simulink model "washout"  (R2018b)
settings: Solver=VariableStepAuto  StartTime=0.0  StopTime=Time(end)  RelTol=1e-3
values from neighbouring files (symbols this model uses):
  Cf = 80000    [init.m]
  Cr = 90000    [init.m]
  dG = 0.05    [init.m]
  g = 9.81    [init.m]
  lf = cog_x*L    (= 0.70125)    [init.m]
  lr = (1-cog_x)*L    (= 2.10375)    [init.m]
  mass = 1905    [init.m]
  Ratio = 10    [init.m]
  rx = 30e-2    (= 0.3)    [init.m]
  swaThreshold = 5    [init.m]
  T0 = 0.3    [init.m]
  TH = 0.1    [init.m]
  TTh = 0.1    [init.m]
  vxThreshold = 0.5    [init.m]
  xC = 0    [init.m]
  xG = 0.01    [init.m]
  yawThreshold = 0.1    [init.m]
undefined symbols (not defined in the file or in its folder): T
libraries: simulink_extras x3, dsparch4 x1
settings Model: Creator=carl  LastModifiedBy=carl

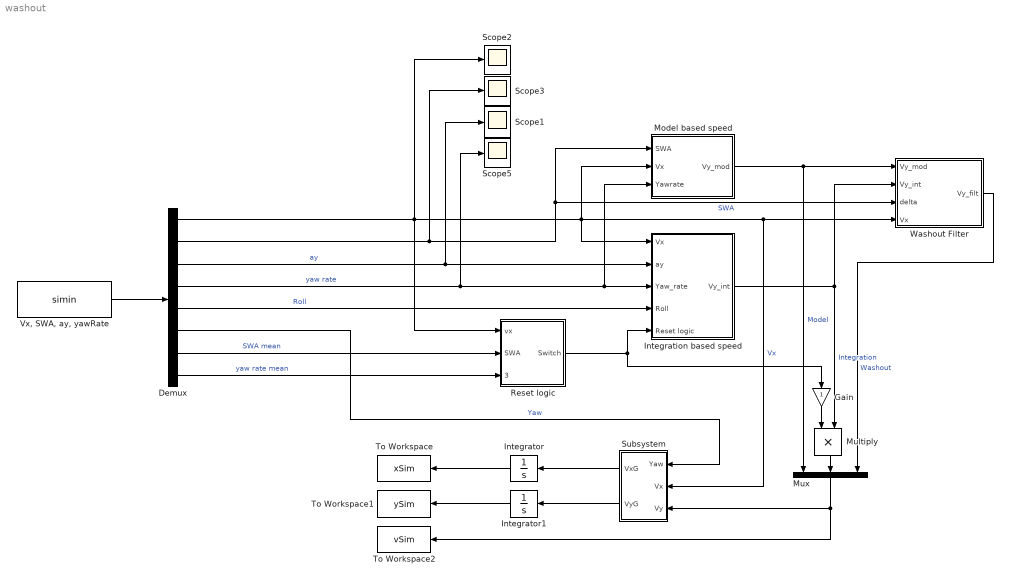
== system washout ==
  Demux : Demux  Outputs=8
  Gain : Gain
  Integration based speed : Subsystem
  Integrator : Integrator
  Integrator1 : Integrator
  Model based speed : Subsystem
  Multiply : Product
  Mux : Mux  Inputs=3
  Reset logic : Subsystem
  Scope{1..3,5} (4 alike) : Scope
  Subsystem : Subsystem
  To Workspace : ToWorkspace  VariableName=xSim  SaveFormat=Timeseries  SampleTime=-1
  To Workspace1 : ToWorkspace  VariableName=ySim  SaveFormat=Timeseries  SampleTime=-1
  To Workspace2 : ToWorkspace  VariableName=vSim  SaveFormat=Timeseries  SampleTime=-1
  "Vx, SWA, ay, yawRate" : FromWorkspace  VariableName=simin  SampleTime=0
  Washout Filter : Subsystem
  wires:
  Demux/3 -> Scope1/1, Integration based speed/2(ay)  "ay"
  Model based speed/1(Vy_mod) -> Mux/1, Washout Filter/1(Vy_mod)  "Model"
  Demux/2 -> Scope3/1, Washout Filter/3(delta), Model based speed/1(SWA)  "SWA"
  Demux/1 -> Reset logic/1(vx), Integration based speed/1(Vx), Washout Filter/4(Vx), Subsystem/2(Vx), Model based speed/2(Vx), Scope2/1  "Vx"
  Integration based speed/1(Vy_int) -> Multiply/2, Washout Filter/2(Vy_int)  "Integration"
  Demux/4 -> Model based speed/3(Yawrate), Integration based speed/3(Yaw_rate), Scope5/1  "yaw rate"
  Washout Filter/1(Vy_filt) -> Mux/3  "Washout"
  Integrator/1 -> To Workspace/1
  "Vx, SWA, ay, yawRate"/1 -> Demux/1
  Integrator1/1 -> To Workspace1/1
  Subsystem/2(VyG) -> Integrator1/1
  Subsystem/1(VxG) -> Integrator/1
  Demux/5 -> Integration based speed/4(Roll)  "Roll"
  Demux/6 -> Subsystem/1(Yaw)  "Yaw"
  Mux/1 -> To Workspace2/1, Subsystem/3(Vy)
  Reset logic/1(Switch) -> Gain/1, Integration based speed/5(Reset logic)
  Multiply/1 -> Mux/2
  Gain/1 -> Multiply/1
  Demux/7 -> Reset logic/2(SWA)  "SWA mean"
  Demux/8 -> Reset logic/3(yawrate)  "yaw rate mean"

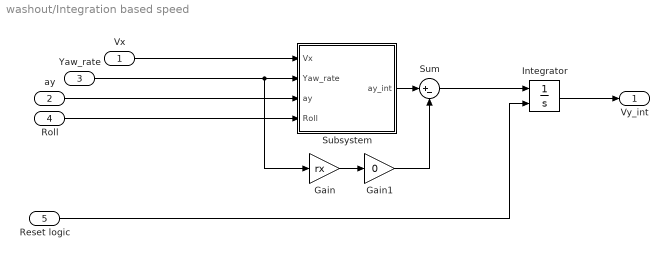
== system washout/Integration based speed ==
  Vx : Inport
  ay : Inport  Port=2
  Yaw_rate : Inport  Port=3
  Roll : Inport  Port=4
  Reset logic : Inport  Port=5
  Gain : Gain  Gain=rx
  Gain1 : Gain  Gain=0
  Integrator : Integrator  ExternalReset=rising
  Subsystem : Subsystem
  Sum : Sum  Inputs=|+-
  Vy_int : Outport
  wires:
  Vx/1 -> Subsystem/1(Vx)
  Yaw_rate/1 -> Gain/1, Subsystem/2(Yaw_rate)
  ay/1 -> Subsystem/3(ay)
  Subsystem/1(ay_int) -> Sum/1
  Roll/1 -> Subsystem/4(Roll)
  Gain/1 -> Gain1/1
  Gain1/1 -> Sum/2
  Sum/1 -> Integrator/1
  Integrator/1 -> Vy_int/1
  Reset logic/1 -> Integrator/2

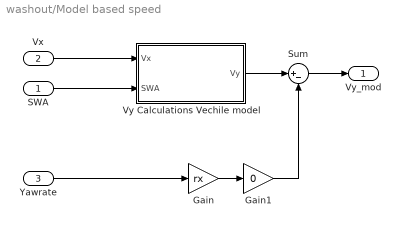
== system washout/Model based speed ==
  SWA : Inport
  Vx : Inport  Port=2
  Yawrate : Inport  Port=3
  Gain : Gain  Gain=rx
  Gain1 : Gain  Gain=0
  Sum : Sum  Inputs=|+-
  Vy Calculations Vechile model : Subsystem
  Vy_mod : Outport
  wires:
  Vx/1 -> Vy Calculations Vechile model/1(Vx)
  Vy Calculations Vechile model/1(Vy) -> Sum/1
  SWA/1 -> Vy Calculations Vechile model/2(SWA)
  Sum/1 -> Vy_mod/1
  Yawrate/1 -> Gain/1
  Gain/1 -> Gain1/1
  Gain1/1 -> Sum/2

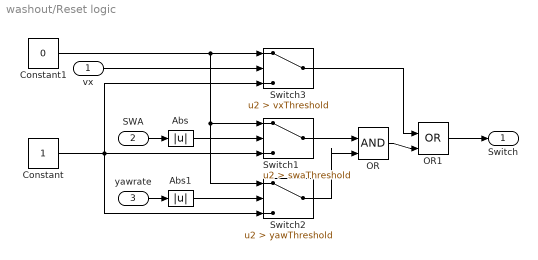
== system washout/Reset logic ==
  vx : Inport
  SWA : Inport  Port=2
  yawrate : Inport  Port=3
  Abs : Abs
  Abs1 : Abs
  Constant : Constant
  Constant1 : Constant  Value=0
  OR : Logic  IconShape=distinctive  AllPortsSameDT=off  OutDataTypeStr=boolean
  OR1 : Logic  Operator=OR  IconShape=distinctive  AllPortsSameDT=off  OutDataTypeStr=boolean
  Switch1 : Switch  Criteria=u2 > Threshold  Threshold=swaThreshold
  Switch2 : Switch  Criteria=u2 > Threshold  Threshold=yawThreshold
  Switch3 : Switch  Criteria=u2 > Threshold  Threshold=vxThreshold
  Switch : Outport
  wires:
  OR1/1 -> Switch/1
  Switch2/1 -> OR/2
  Constant/1 -> Switch1/3, Switch3/3, Switch2/3
  Abs/1 -> Switch1/2
  SWA/1 -> Abs/1
  yawrate/1 -> Abs1/1
  OR/1 -> OR1/2
  Switch1/1 -> OR/1
  Switch3/1 -> OR1/1
  Constant1/1 -> Switch1/1, Switch2/1, Switch3/1
  Abs1/1 -> Switch2/2
  vx/1 -> Switch3/2

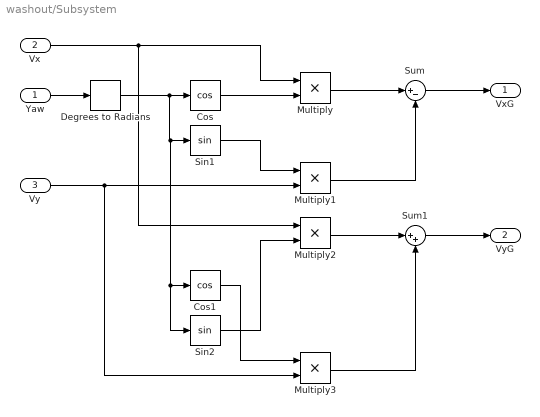
== system washout/Subsystem ==
  Yaw : Inport
  Vx : Inport  Port=2
  Vy : Inport  Port=3
  Cos : Trigonometry  Operator=cos
  Cos1 : Trigonometry  Operator=cos
  Degrees to Radians : simulink_extras/Transformations/Degrees to Radians
  Multiply{,1..3} (4 alike) : Product
  Sin1 : Trigonometry
  Sin2 : Trigonometry
  Sum : Sum  Inputs=|+-
  Sum1 : Sum  Inputs=|++
  VxG : Outport
  VyG : Outport  Port=2
  wires:
  Multiply/1 -> Sum/1
  Cos/1 -> Multiply/2
  Sin1/1 -> Multiply1/1
  Multiply1/1 -> Sum/2
  Sum/1 -> VxG/1
  Multiply2/1 -> Sum1/1
  Vx/1 -> Multiply2/1, Multiply/1
  Multiply3/1 -> Sum1/2
  Vy/1 -> Multiply1/2, Multiply3/2
  Sum1/1 -> VyG/1
  Sin2/1 -> Multiply2/2
  Cos1/1 -> Multiply3/1
  Yaw/1 -> Degrees to Radians/1
  Degrees to Radians/1 -> Sin2/1, Cos1/1, Sin1/1, Cos/1

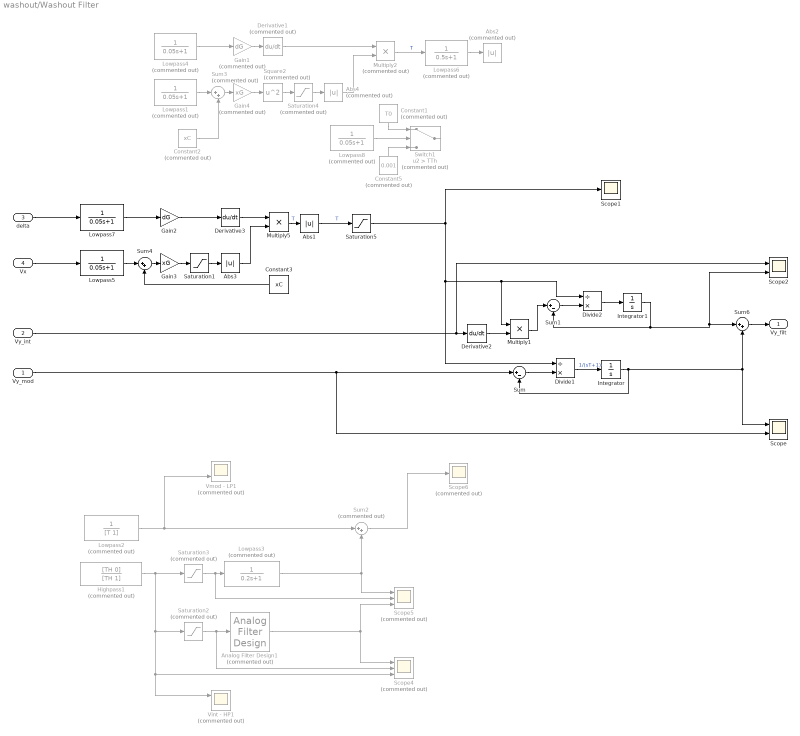
== system washout/Washout Filter ==
  Vy_mod : Inport
  Vy_int : Inport  Port=2
  delta : Inport  Port=3
  Vx : Inport  Port=4
  Abs1 : Abs
  Abs2 : Abs  Commented=on
  Abs3 : Abs
  Abs4 : Abs  Commented=on
  Analog Filter Design1 : dsparch4/Analog Filter Design  Commented=on  method=Butterworth  filttype=Lowpass  N=7  Wlo=8  Whi=80  Rp=2  Rs=40
  Constant1 : Constant  Commented=on  Value=T0
  Constant2 : Constant  Commented=on  Value=xC
  Constant3 : Constant  Value=xC
  Constant5 : Constant  Commented=on  Value=0.001
  Derivative1 : Derivative  Commented=on
  Derivative2 : Derivative
  Derivative3 : Derivative
  Divide1 : Product  Inputs=/*
  Divide2 : Product  Inputs=/*
  Gain1 : Gain  Commented=on  Gain=dG
  Gain2 : Gain  Gain=dG
  Gain3 : Gain  Gain=xG
  Gain4 : Gain  Commented=on  Gain=xG
  Highpass1 : TransferFcn  Commented=on  Numerator=[TH 0]  Denominator=[TH 1]
  Integrator : Integrator
  Integrator1 : Integrator
  Lowpass1 : TransferFcn  Commented=on  Denominator=[0.05 1]
  Lowpass2 : TransferFcn  Commented=on  Denominator=[T 1]
  Lowpass3 : TransferFcn  Commented=on  Denominator=[0.2 1]
  Lowpass4 : TransferFcn  Commented=on  Denominator=[0.05 1]
  Lowpass5 : TransferFcn  Denominator=[0.05 1]
  Lowpass6 : TransferFcn  Commented=on  Denominator=[0.5 1]
  Lowpass7 : TransferFcn  Denominator=[0.05 1]
  Lowpass8 : TransferFcn  Commented=on  Denominator=[0.05 1]
  Multiply1 : Product
  Multiply2 : Product  Commented=on
  Multiply5 : Product
  Saturation1 : Saturate  UpperLimit=2  LowerLimit=0
  Saturation2 : Saturate  Commented=on  UpperLimit=1  LowerLimit=-1
  Saturation3 : Saturate  Commented=on  UpperLimit=1  LowerLimit=-1
  Saturation4 : Saturate  Commented=on  UpperLimit=2  LowerLimit=0
  Saturation5 : Saturate  UpperLimit=T0  LowerLimit=0.01
  Scope : Scope  NumInputPorts=2
  Scope1 : Scope
  Scope2 : Scope  NumInputPorts=2
  Scope4 : Scope  Commented=on  NumInputPorts=3
  Scope5 : Scope  Commented=on  NumInputPorts=3
  Scope6 : Scope  Commented=on
  Square2 : Math  Commented=on  Operator=square  SaturateOnIntegerOverflow=on
  Sum : Sum  Inputs=|+-
  Sum1 : Sum  Inputs=|+-
  Sum2 : Sum  Commented=on  Inputs=|++
  Sum3 : Sum  Commented=on  Inputs=|++
  Sum4 : Sum  Inputs=|++
  Sum6 : Sum  Inputs=|++
  Switch1 : Switch  Commented=on  Criteria=u2 > Threshold  Threshold=TTh
  Vint - HP1 : Scope  Commented=on  NumInputPorts=2
  Vmod - LP1 : Scope  Commented=on  NumInputPorts=2
  Vy_filt : Outport
  wires:
  Saturation3/1 -> Lowpass3/1, Scope5/2
  Saturation2/1 -> Analog Filter Design1/1, Scope4/2
  Analog Filter Design1/1 -> Scope5/3, Scope4/1
  Lowpass3/1 -> Sum2/2, Scope5/1
  Lowpass2/1 -> Sum2/1, Vmod - LP1/2
  Sum2/1 -> Scope6/1
  Highpass1/1 -> Vint - HP1/1, Scope4/3, Saturation2/1, Saturation3/1
  Constant3/1 -> Sum4/2
  Sum4/1 -> Gain3/1
  Saturation1/1 -> Abs3/1
  Gain3/1 -> Saturation1/1
  Multiply5/1 -> Abs1/1  "T"
  Abs3/1 -> Multiply5/2
  Lowpass5/1 -> Sum4/1
  Derivative3/1 -> Multiply5/1
  Lowpass7/1 -> Gain2/1
  Gain2/1 -> Derivative3/1
  Gain1/1 -> Derivative1/1
  Lowpass4/1 -> Gain1/1
  Derivative1/1 -> Multiply2/1
  Lowpass6/1 -> Abs2/1
  Lowpass1/1 -> Sum3/1
  Abs4/1 -> Multiply2/2
  Multiply2/1 -> Lowpass6/1  "T"
  Gain4/1 -> Square2/1
  Square2/1 -> Saturation4/1
  Saturation4/1 -> Abs4/1
  Sum3/1 -> Gain4/1
  Constant2/1 -> Sum3/2
  Abs1/1 -> Saturation5/1  "T"
  delta/1 -> Lowpass7/1
  Vx/1 -> Lowpass5/1
  Derivative2/1 -> Multiply1/2
  Vy_int/1 -> Scope2/1, Derivative2/1
  Vy_mod/1 -> Sum/1, Scope/2
  Sum6/1 -> Vy_filt/1
  Sum/1 -> Divide1/2
  Divide1/1 -> Integrator/1  "1/(sT+1)"
  Integrator/1 -> Scope/1, Sum6/2, Sum/2
  Multiply1/1 -> Sum1/1
  Sum1/1 -> Divide2/2
  Divide2/1 -> Integrator1/1
  Integrator1/1 -> Scope2/2, Sum6/1, Sum1/2
  Lowpass8/1 -> Switch1/2
  Constant5/1 -> Switch1/3
  Constant1/1 -> Switch1/1
  Saturation5/1 -> Divide1/1, Multiply1/1, Divide2/1, Scope1/1

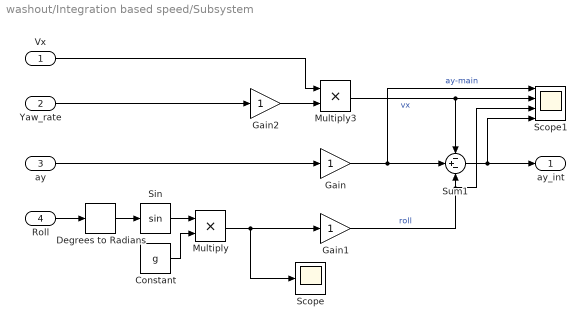
== system washout/Integration based speed/Subsystem ==
  Vx : Inport
  Yaw_rate : Inport  Port=2
  ay : Inport  Port=3
  Roll : Inport  Port=4
  Constant : Constant  Value=g
  Degrees to Radians : simulink_extras/Transformations/Degrees to Radians
  Gain : Gain
  Gain1 : Gain
  Gain2 : Gain
  Multiply : Product
  Multiply3 : Product
  Scope : Scope
  Scope1 : Scope  NumInputPorts=4
  Sin : Trigonometry
  Sum1 : Sum  Inputs=-+-
  ay_int : Outport
  wires:
  Multiply3/1 -> Sum1/1, Scope1/2  "vx"
  Vx/1 -> Multiply3/1
  Sum1/1 -> Scope1/4, ay_int/1
  Yaw_rate/1 -> Gain2/1
  Sin/1 -> Multiply/1
  Roll/1 -> Degrees to Radians/1
  Constant/1 -> Multiply/2
  Degrees to Radians/1 -> Sin/1
  Multiply/1 -> Scope/1, Gain1/1
  ay/1 -> Gain/1
  Gain/1 -> Scope1/1, Sum1/2  "ay-main"
  Gain1/1 -> Scope1/3, Sum1/3  "roll"
  Gain2/1 -> Multiply3/2

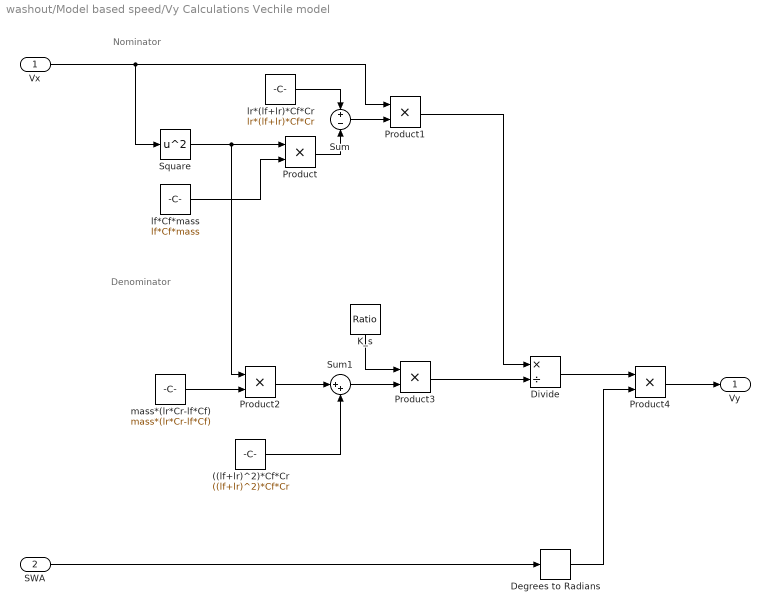
== system washout/Model based speed/Vy Calculations Vechile model ==
  note: Nominator
  note: Denominator
  Vx : Inport
  SWA : Inport  Port=2
  ((lf+lr)^2)*Cf*Cr : Constant  Value=((lf+lr)^2)*Cf*Cr
  Degrees to Radians : simulink_extras/Transformations/Degrees to Radians
  Divide : Product  Inputs=*/
  K_s : Constant  Value=Ratio
  Product{,1..4} (5 alike) : Product
  Square : Math  Operator=square  RndMeth=Zero  SaturateOnIntegerOverflow=on
  Sum : Sum  Inputs=+-
  Sum1 : Sum  Inputs=|++
  lf*Cf*mass : Constant  Value=lf*Cf*mass
  lr*(lf+lr)*Cf*Cr : Constant  Value=lr*(lf+lr)*Cf*Cr
  mass*(lr*Cr-lf*Cf) : Constant  Value=mass*(lr*Cr-lf*Cf)
  Vy : Outport
  wires:
  Product1/1 -> Divide/1
  Product3/1 -> Divide/2
  Vx/1 -> Product1/1, Square/1
  lr*(lf+lr)*Cf*Cr/1 -> Sum/1
  Sum/1 -> Product1/2
  Product/1 -> Sum/2
  Square/1 -> Product2/1, Product/1
  lf*Cf*mass/1 -> Product/2
  Product2/1 -> Sum1/1
  mass*(lr*Cr-lf*Cf)/1 -> Product2/2
  Sum1/1 -> Product3/2
  ((lf+lr)^2)*Cf*Cr/1 -> Sum1/2
  Divide/1 -> Product4/1
  Product4/1 -> Vy/1
  K_s/1 -> Product3/1
  SWA/1 -> Degrees to Radians/1
  Degrees to Radians/1 -> Product4/2
